simulink library "quat2EulerAng_ul"  (R2018b)
settings: Solver=VariableStepAuto  StartTime=0.0  StopTime=10.0  RelTol=1e-3
settings Model: Creator=mcobb  LastModifiedBy=mcobb

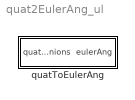
== system quat2EulerAng_ul ==
  quatToEulerAng : Subsystem

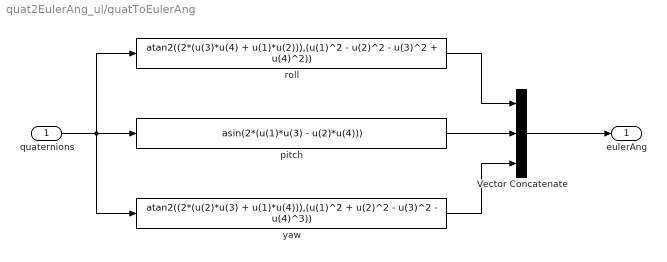
== system quat2EulerAng_ul/quatToEulerAng ==
  quaternions : Inport
  Vector Concatenate : Concatenate  NumInputs=3
  pitch : Fcn  Expr=asin(2*(u(1)*u(3) - u(2)*u(4)))
  roll : Fcn  Expr=atan2((2*(u(3)*u(4) + u(1)*u(2))),(u(1)^2 - u(2)^2 - u(3)^2 + u(4)^2))
  yaw : Fcn  Expr=atan2((2*(u(2)*u(3) + u(1)*u(4))),(u(1)^2 + u(2)^2 - u(3)^2 - u(4)^3))
  eulerAng : Outport  PortDimensions=[3,1]
  wires:
  quaternions/1 -> yaw/1, roll/1, pitch/1
  pitch/1 -> Vector Concatenate/2
  roll/1 -> Vector Concatenate/1
  yaw/1 -> Vector Concatenate/3
  Vector Concatenate/1 -> eulerAng/1
